simulink model "hw5"  (Simulink 7.3)
settings: Solver=ode45  StartTime=0.0  StopTime=5  RelTol=1e-3
settings Model: Creator=m134506  LastModifiedBy=m134506

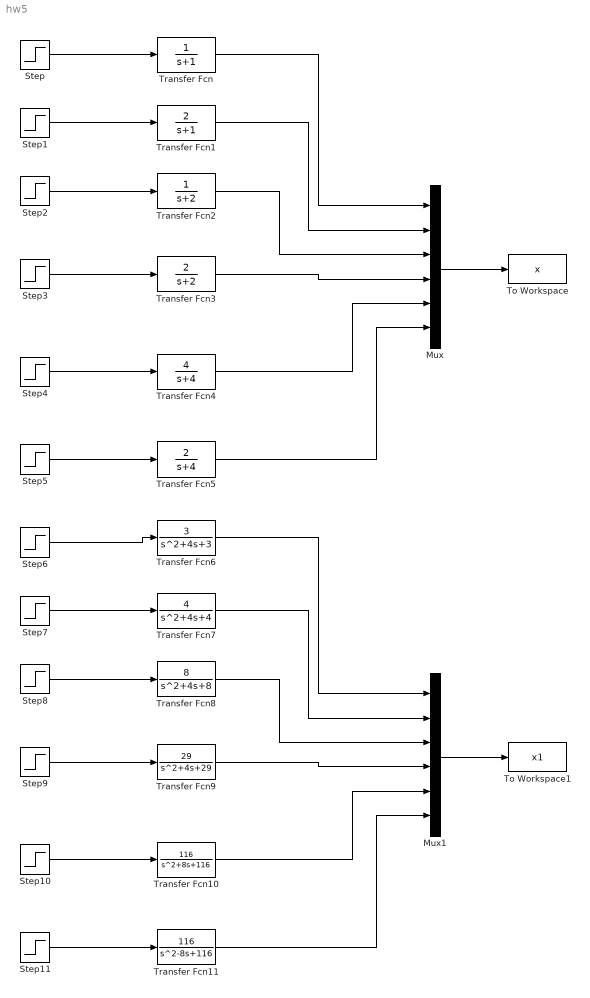
== system hw5 ==
  Mux : Mux  Inputs=6
  Mux1 : Mux  Inputs=6
  Step{,1..11} (12 alike) : Step  Time=0  SampleTime=0
  To Workspace : ToWorkspace  VariableName=x  SampleTime=-1  SaveFormat=Array
  To Workspace1 : ToWorkspace  VariableName=x1  SampleTime=-1  SaveFormat=Array
  Transfer Fcn : TransferFcn  Denominator=[1 1]
  Transfer Fcn1 : TransferFcn  Numerator=2  Denominator=[1 1]
  Transfer Fcn10 : TransferFcn  Numerator=116  Denominator=[1 8 116]
  Transfer Fcn11 : TransferFcn  Numerator=116  Denominator=[1 -8 116]
  Transfer Fcn2 : TransferFcn  Denominator=[1 2]
  Transfer Fcn3 : TransferFcn  Numerator=2  Denominator=[1 2]
  Transfer Fcn4 : TransferFcn  Numerator=4  Denominator=[1 4]
  Transfer Fcn5 : TransferFcn  Numerator=2  Denominator=[1 4]
  Transfer Fcn6 : TransferFcn  Numerator=3  Denominator=[1 4 3]
  Transfer Fcn7 : TransferFcn  Numerator=4  Denominator=[1 4 4]
  Transfer Fcn8 : TransferFcn  Numerator=8  Denominator=[1 4 8]
  Transfer Fcn9 : TransferFcn  Numerator=29  Denominator=[1 4 29]
  wires:
  Step/1 -> Transfer Fcn/1
  Step1/1 -> Transfer Fcn1/1
  Step2/1 -> Transfer Fcn2/1
  Step3/1 -> Transfer Fcn3/1
  Step4/1 -> Transfer Fcn4/1
  Step5/1 -> Transfer Fcn5/1
  Transfer Fcn/1 -> Mux/1
  Transfer Fcn5/1 -> Mux/6
  Transfer Fcn4/1 -> Mux/5
  Transfer Fcn3/1 -> Mux/4
  Transfer Fcn2/1 -> Mux/3
  Transfer Fcn1/1 -> Mux/2
  Mux/1 -> To Workspace/1
  Step6/1 -> Transfer Fcn6/1
  Step7/1 -> Transfer Fcn7/1
  Step8/1 -> Transfer Fcn8/1
  Step9/1 -> Transfer Fcn9/1
  Step10/1 -> Transfer Fcn10/1
  Step11/1 -> Transfer Fcn11/1
  Transfer Fcn6/1 -> Mux1/1
  Transfer Fcn11/1 -> Mux1/6
  Transfer Fcn10/1 -> Mux1/5
  Transfer Fcn9/1 -> Mux1/4
  Transfer Fcn8/1 -> Mux1/3
  Transfer Fcn7/1 -> Mux1/2
  Mux1/1 -> To Workspace1/1
